simulink model "CSTR_RL_eval"  (R2021a)
settings: Solver=FixedStepAuto  StartTime=0.0  StopTime=T  FixedStep=Ts  RelTol=1e-3
InitFcn:
  | seed = randi(10000);
StartFcn:
  | seed = randi(10000);
undefined symbols (not defined in the file): change_freq, isTerminate, Ts, x0
libraries: simulink x3, sharedTrackingLibrary x1, rllib x1
settings Model: Creator=The MathWorks, Inc.  LastModifiedBy=jiaya
settings SolverCC: AlgebraicLoopSolver=TrustRegion
settings DataIOCC: ReturnWorkspaceOutputs=off
settings DebuggingCC: SFMachineParentedDataDiag=warning  ArithmeticOperatorsInVariantConditions=warning
settings SFSimCC: SimUseLocalCustomCode=off  CustomCodeUndefinedFunction=UseInterfaceOnly
settings RTWCC: RTWUseLocalCustomCode=off

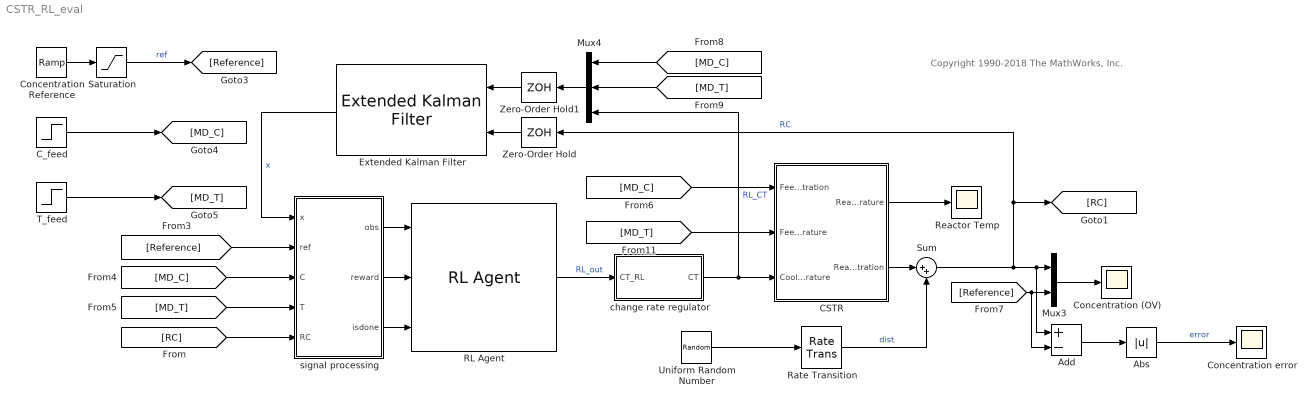
== system CSTR_RL_eval ==
  note: Copyright 1990-2018 The MathWorks, Inc.
  Abs : Abs
  Add : Sum  Inputs=+-
  CSTR : Subsystem
  C_feed : Step  Time=10  Before=10  After=10.3  SampleTime=0
  Concentration Reference : simulink/Sources/Ramp  slope=-0.45  start=1  InitialOutput=x0(2)
  Concentration (OV) : Scope
  Concentration error : Scope
  Extended Kalman Filter : sharedTrackingLibrary/Extended Kalman Filter  StateTransitionFcn=exocstrStateFcnDT  HasStateTransitionJacobianFcn=off  HasAdditiveProcessNoise=Additive  ProcessNoise=1e-3  HasTimeVaryingProcessNoise=off  HasStateTransitionFcnExtraArgument=1  InitialState=x0  InitialStateCovariance=1e-3  MeasurementFcn1=exocstrMeasFcn  HasMeasurementJacobianFcn1=off  HasMeasurementEnablePort1=off  HasAdditiveMeasurementNoise1=Additive  MeasurementNoise1=1e-3  HasTimeVaryingMeasurementNoise1=off  HasMeasurementFcnExtraArgument1=0  MeasurementFcn2=myMeasurementFcn  HasMeasurementJacobianFcn2=off  HasMeasurementEnablePort2=off  HasAdditiveMeasurementNoise2=Additive  MeasurementNoise2=1  HasTimeVaryingMeasurementNoise2=off  HasMeasurementFcnExtraArgument2=0  MeasurementFcn3=myMeasurementFcn  HasMeasurementJacobianFcn3=off  HasMeasurementEnablePort3=off  HasAdditiveMeasurementNoise3=Additive  MeasurementNoise3=1  HasTimeVaryingMeasurementNoise3=off  HasMeasurementFcnExtraArgument3=0  MeasurementFcn4=myMeasurementFcn  HasMeasurementJacobianFcn4=off  HasMeasurementEnablePort4=off  HasAdditiveMeasurementNoise4=Additive  MeasurementNoise4=1  HasTimeVaryingMeasurementNoise4=off  HasMeasurementFcnExtraArgument4=0  MeasurementFcn5=myMeasurementFcn  HasMeasurementJacobianFcn5=off  HasMeasurementEnablePort5=off  HasAdditiveMeasurementNoise5=Additive  MeasurementNoise5=1  HasTimeVaryingMeasurementNoise5=off  HasMeasurementFcnExtraArgument5=0  EnableMultirate=off  StateTransitionFcnSampleTime=1  MeasurementFcn1SampleTime=1  MeasurementFcn2SampleTime=1  MeasurementFcn3SampleTime=1  MeasurementFcn4SampleTime=1  MeasurementFcn5SampleTime=1  UseCurrentEstimator=on  OutputStateCovariance=off  DataType=double  SampleTime=Ts  NumberOfMeasurements=1
      settings: SourceProductBaseCode=CT,DR,TF,ID,LP,NV,AR,RO,RR,UV,VE
  Mux3 : Mux  Inputs=2
  Mux4 : Mux  Inputs=3
  RL Agent : rllib/RL Agent  Agent=agent  ExternalActionAsInput=off  ProvideCumRwd=off  TreatAsDirectFeedthrough=on
  Rate Transition : RateTransition  OutPortSampleTime=Ts
  Reactor Temp : Scope
  Saturation : Saturate  UpperLimit=10  LowerLimit=2
  Sum : Sum  Inputs=|++
  T_feed : Step  Time=20  Before=298.15  After=298.15  SampleTime=301
  Uniform Random Number : UniformRandomNumber  Minimum=0  Maximum=0.5  Seed=seed  SampleTime=change_freq
  Zero-Order Hold : ZeroOrderHold  SampleTime=Ts
  Zero-Order Hold1 : ZeroOrderHold  SampleTime=Ts
  change rate regulator : Subsystem
  signal processing : Subsystem
  wires:
  RL Agent/1 -> change rate regulator/1(CT_RL)  "RL_out"
  CSTR/1(Reactor Temperature) -> Reactor Temp/1
  Concentration Reference/1 -> Saturation/1
  Mux3/1 -> Concentration (OV)/1
  Extended Kalman Filter/1 -> signal processing/1(x)  "x"
  Zero-Order Hold/1 -> Extended Kalman Filter/2
  Mux4/1 -> Zero-Order Hold1/1
  Zero-Order Hold1/1 -> Extended Kalman Filter/1
  Sum/1 -> Add/1, Mux3/1, Zero-Order Hold/1, [RC]  "RC"
  Rate Transition/1 -> Sum/2  "dist"
  CSTR/2(Reactor Concentration) -> Sum/1
  Saturation/1 -> [Reference]  "ref"
  [Reference] -> signal processing/2(ref)
  C_feed/1 -> [MD_C]
  T_feed/1 -> [MD_T]
  [MD_C] -> signal processing/3(C)
  [MD_T] -> signal processing/4(T)
  [MD_C] -> CSTR/1(Feed Concentration)
  [Reference] -> Add/2, Mux3/2
  [MD_C] -> Mux4/1
  [MD_T] -> Mux4/2
  [MD_T] -> CSTR/2(Feed Temperature)
  Uniform Random Number/1 -> Rate Transition/1
  signal processing/1(obs) -> RL Agent/1
  signal processing/2(reward) -> RL Agent/2
  signal processing/3(isdone) -> RL Agent/3
  change rate regulator/1("CT ") -> Mux4/3, CSTR/3(Coolant Temperature)  "RL_CT"
  [RC] -> signal processing/5(RC)
  Add/1 -> Abs/1
  Abs/1 -> Concentration error/1  "error"

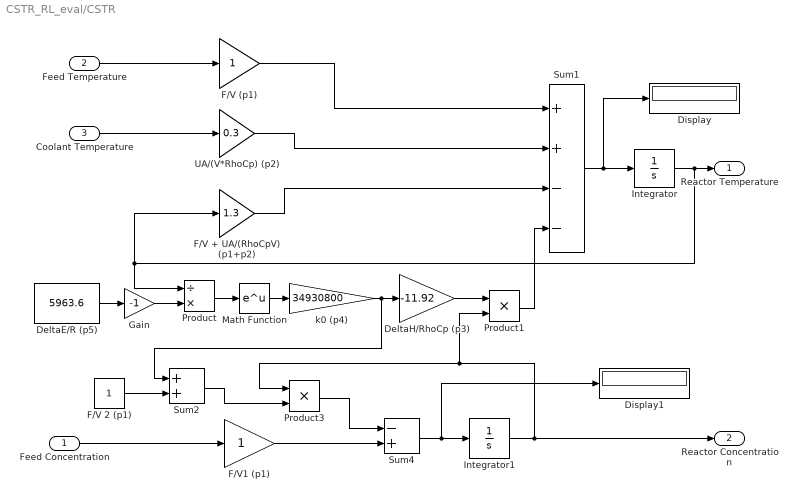
== system CSTR_RL_eval/CSTR ==
  Feed Concentration : Inport
  Feed Temperature : Inport  Port=2
  Coolant Temperature : Inport  Port=3
  DeltaE/R (p5) : Constant  Value=5963.6
  DeltaH/RhoCp (p3) : Gain  Gain=-11.92  SaturateOnIntegerOverflow=on  OutDataTypeStr=Inherit: Same as input  ParamDataTypeStr=Inherit: Same as input
  Display : Display
  Display1 : Display
  F/V (p1) : Gain  SaturateOnIntegerOverflow=on  OutDataTypeStr=Inherit: Same as input  ParamDataTypeStr=Inherit: Same as input
  F/V + UA/(RhoCpV) (p1+p2) : Gain  Gain=1.3  SaturateOnIntegerOverflow=on  OutDataTypeStr=Inherit: Same as input  ParamDataTypeStr=Inherit: Same as input
  F/V 2 (p1) : Constant
  F/V1 (p1) : Gain  SaturateOnIntegerOverflow=on  OutDataTypeStr=Inherit: Same as input  ParamDataTypeStr=Inherit: Same as input
  Gain : Gain  Gain=-1
  Integrator : Integrator  InitialCondition=x0(1)  LimitOutput=on  LowerSaturationLimit=0
  Integrator1 : Integrator  InitialCondition=x0(2)  LimitOutput=on  LowerSaturationLimit=0
  Math Function : Math  SignedPower=on  SaturateOnIntegerOverflow=on
  Product : Product  Inputs=/*  InputSameDT=on  RndMeth=Zero  SaturateOnIntegerOverflow=on  OutDataTypeStr=Inherit: Same as first input
  Product1 : Product  InputSameDT=on  RndMeth=Zero  SaturateOnIntegerOverflow=on  OutDataTypeStr=Inherit: Same as first input
  Product3 : Product  InputSameDT=on  RndMeth=Zero  SaturateOnIntegerOverflow=on  OutDataTypeStr=Inherit: Same as first input
  Sum1 : Sum  Inputs=++--  InputSameDT=on  SaturateOnIntegerOverflow=on  OutDataTypeStr=Inherit: Same as first input
  Sum2 : Sum  InputSameDT=on  SaturateOnIntegerOverflow=on  OutDataTypeStr=Inherit: Same as first input
  Sum4 : Sum  Inputs=-+  InputSameDT=on  SaturateOnIntegerOverflow=on  OutDataTypeStr=Inherit: Same as first input
  UA/(V*RhoCp) (p2) : Gain  Gain=0.3  SaturateOnIntegerOverflow=on  OutDataTypeStr=Inherit: Same as input  ParamDataTypeStr=Inherit: Same as input
  k0 (p4) : Gain  Gain=34930800  SaturateOnIntegerOverflow=on  OutDataTypeStr=Inherit: Same as input  ParamDataTypeStr=Inherit: Same as input
  Reactor Temperature : Outport  VectorParamsAs1DForOutWhenUnconnected=off
  Reactor Concentration : Outport  Port=2  VectorParamsAs1DForOutWhenUnconnected=off
  wires:
  F/V (p1)/1 -> Sum1/1
  Sum1/1 -> Display/1, Integrator/1
  Integrator/1 -> Product/1, F/V + UA/(RhoCpV) (p1+p2)/1, Reactor Temperature/1
  UA/(V*RhoCp) (p2)/1 -> Sum1/2
  F/V + UA/(RhoCpV) (p1+p2)/1 -> Sum1/3
  Product/1 -> Math Function/1
  Math Function/1 -> k0 (p4)/1
  DeltaH/RhoCp (p3)/1 -> Product1/1
  Product1/1 -> Sum1/4
  k0 (p4)/1 -> DeltaH/RhoCp (p3)/1, Sum2/1
  DeltaE/R (p5)/1 -> Gain/1
  Product3/1 -> Sum4/1
  Sum4/1 -> Display1/1, Integrator1/1
  Integrator1/1 -> Product1/2, Product3/1, Reactor Concentration/1
  F/V 2 (p1)/1 -> Sum2/2
  F/V1 (p1)/1 -> Sum4/2
  Feed Temperature/1 -> F/V (p1)/1
  Feed Concentration/1 -> F/V1 (p1)/1
  Coolant Temperature/1 -> UA/(V*RhoCp) (p2)/1
  Sum2/1 -> Product3/2
  Gain/1 -> Product/2

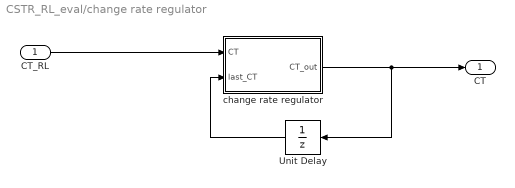
== system CSTR_RL_eval/change rate regulator ==
  CT_RL : Inport
  Unit Delay : UnitDelay  InitialCondition=300  SampleTime=-1  HasFrameUpgradeWarning=on
  change rate regulator : MATLAB Function  TreatAsAtomicUnit=on
  "CT " : Outport
  wires:
  CT_RL/1 -> change rate regulator/1(CT)
  Unit Delay/1 -> change rate regulator/2(last_CT)
  change rate regulator/1(CT_out) -> Unit Delay/1, "CT "/1

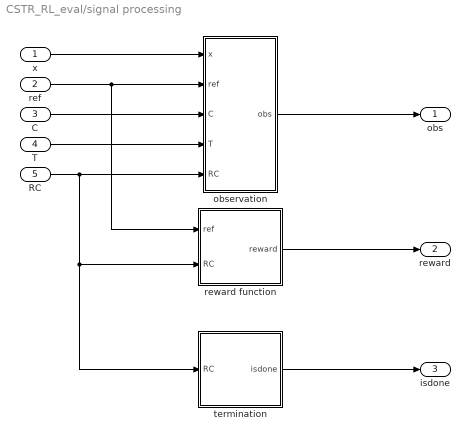
== system CSTR_RL_eval/signal processing ==
  x : Inport
  ref : Inport  Port=2
  C : Inport  Port=3
  T : Inport  Port=4
  RC : Inport  Port=5
  observation : Subsystem
  reward function : Subsystem
  termination : Subsystem
  obs : Outport
  reward : Outport  Port=2
  isdone : Outport  Port=3
  wires:
  x/1 -> observation/1(x)
  ref/1 -> reward function/1(ref), observation/2(ref)
  C/1 -> observation/3(C)
  T/1 -> observation/4(T)
  observation/1(obs) -> obs/1
  reward function/1(reward) -> reward/1
  termination/1(isdone) -> isdone/1
  RC/1 -> termination/1(RC), reward function/2(RC), observation/5(RC)

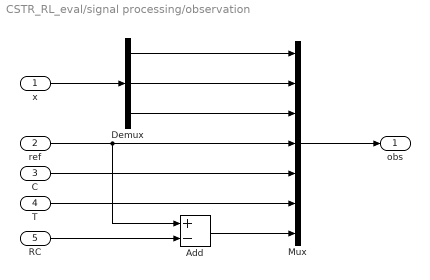
== system CSTR_RL_eval/signal processing/observation ==
  x : Inport
  ref : Inport  Port=2
  C : Inport  Port=3
  T : Inport  Port=4
  RC : Inport  Port=5
  Add : Sum  Inputs=+-
  Demux : Demux  Outputs=3
  Mux : Mux  Inputs=7
  obs : Outport
  wires:
  x/1 -> Demux/1
  Mux/1 -> obs/1
  Demux/1 -> Mux/1
  Demux/2 -> Mux/2
  Demux/3 -> Mux/3
  ref/1 -> Add/1, Mux/4
  C/1 -> Mux/5
  T/1 -> Mux/6
  RC/1 -> Add/2
  Add/1 -> Mux/7

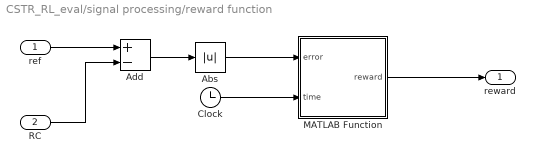
== system CSTR_RL_eval/signal processing/reward function ==
  ref : Inport
  RC : Inport  Port=2
  Abs : Abs
  Add : Sum  Inputs=+-
  Clock : Clock
  MATLAB Function : MATLAB Function  TreatAsAtomicUnit=on
  reward : Outport
  wires:
  ref/1 -> Add/1
  RC/1 -> Add/2
  Add/1 -> Abs/1
  MATLAB Function/1(reward) -> reward/1
  Abs/1 -> MATLAB Function/1(error)
  Clock/1 -> MATLAB Function/2(time)

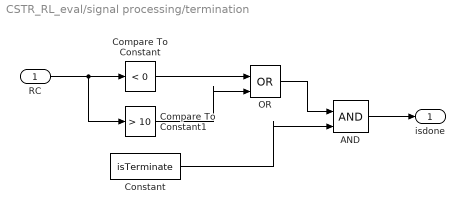
== system CSTR_RL_eval/signal processing/termination ==
  RC : Inport
  AND : Logic  IconShape=distinctive  AllPortsSameDT=off  OutDataTypeStr=boolean
  Compare To Constant : simulink/Logic and Bit Operations/Compare To Constant  relop=<  const=0  OutDataTypeStr=boolean
  Compare To Constant1 : simulink/Logic and Bit Operations/Compare To Constant  relop=>  const=10  OutDataTypeStr=boolean
  Constant : Constant  Value=isTerminate
  OR : Logic  Operator=OR  IconShape=distinctive  AllPortsSameDT=off  OutDataTypeStr=boolean
  isdone : Outport
  wires:
  RC/1 -> Compare To Constant1/1, Compare To Constant/1
  Compare To Constant/1 -> OR/1
  Compare To Constant1/1 -> OR/2
  AND/1 -> isdone/1
  OR/1 -> AND/1
  Constant/1 -> AND/2

== matlab function CSTR_RL_eval/signal processing/reward function/MATLAB Function ==
  data: error input; reward output; time input
function reward = fcn(error, time)

pos = exp(-error);
neg = -tanh(error/1.5);

if error < 1.5
    bonus = 1;
else
    bonus = 0;
end

reward = 3*pos + 2*neg + bonus;

% if time < 15
%     reward = -0.1*tanh(error/1.5);
% else
%     reward = -5*tanh(error*1.5);
% end
% 
% if error < 1
%     reward = reward + 10;
% else
%     reward = reward - 1;
% end

== matlab function CSTR_RL_eval/change rate regulator/change rate regulator ==
  data: CT input; CT_out output; last_CT input
function CT_out = fcn(CT, last_CT)

if CT - last_CT > 5
    CT_out = last_CT + 5;
    
elseif CT - last_CT < -5
    CT_out = last_CT - 5;
    
else
    CT_out = CT;
end
